simulink model "REALIZE_DISCRETE_LOOP_FILTER_L_z_WITHOUT_DELAY"  (R2025b)
settings: Solver=VariableStepAuto  StartTime=0.0  StopTime=100  RelTol=1e-3
libraries: dspsrcs4 x1
settings Model: Creator=Team_33  LastModifiedBy=k2vas

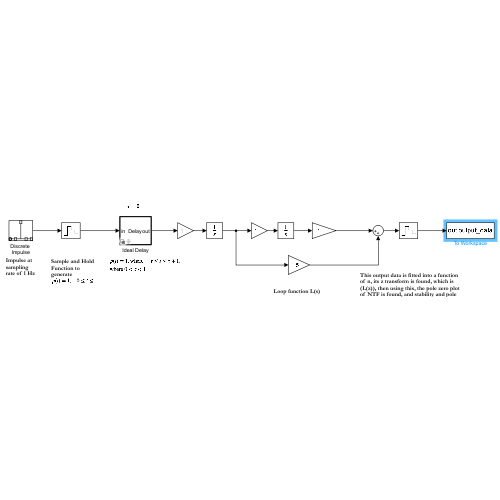
[thumbnail: Simulink's stored preview of the top-level diagram]
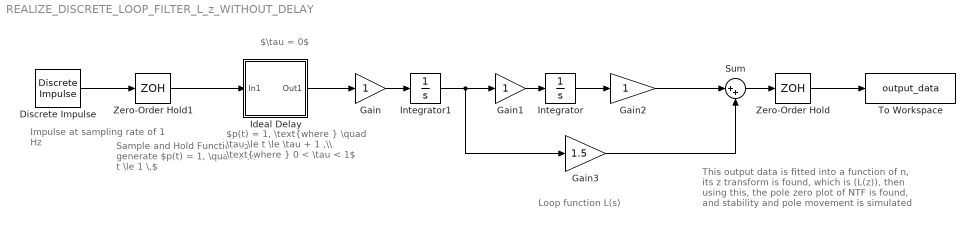
== system REALIZE_DISCRETE_LOOP_FILTER_L_z_WITHOUT_DELAY ==
  note: $\tau = 0$
  note: Sample and Hold Function to generate
      | $p(t) = 1, \quad 0 \le t \le 1 \,$
  note: $p(t) = 1, \text{where } \quad \tau \le t \le \tau + 1 ,\\ \text{where } 0 < \tau < 1$
  note: Impulse at sampling rate of 1 Hz
  note: Loop function L(s)
  note: This output data is fitted into a function of n, its z transform is found, which is (L(z)), then using this, the pole zero plot of NTF is found, and stability and pole movement is simulated
  Discrete Impulse : dspsrcs4/Discrete  Impulse  SFcnStateName=COUNT  Delay=0  SampleTime=1  FrameSample=1  OutputFrames=off  dataType=double  isSigned=on  wordLen=16  udDataType=sfix(16)  fracBitsMode=Best precision  numFracBits=15  OutDataTypeStr=double  LastOutDataTypeStr=double
      settings: SFcnIsStateOwnerBlock=on
  Gain : Gain
  Gain1 : Gain
  Gain2 : Gain
  Gain3 : Gain  Gain=1.5
  Ideal Delay : Subsystem  Variant=on  VariantControlMode=label  LabelModeActiveChoice=delayOFF  mask{eld=0, ts=1}
      mask prompts: eld "Excess delay"; ts "Sampling period"
      mask init:
      | eld = get_param(gcb, 'value@eld');
      |     if eld == 0
      |         set_param(gcb, 'LabelModeActiveChoice', 'delayOFF');
      |     else
      |         set_param(gcb, 'LabelModeActiveChoice', 'delayON');
      |     end
      mask Callback eld:
      | eld = get_param(gcb, 'value@eld');
      |     if eld == 0
      |         set_param(gcb, 'LabelModeActiveChoice', 'delayOFF');
      |     else
      |         set_param(gcb, 'LabelModeActiveChoice', 'delayON');
      |     end
      mask DialogControl DescTextVar Prompt: Ideal delay block (time delay = eld * Ts).
      mask Display:
      | plot([0 1 1 0 0], [0 0 1 1 0]);
      | text(0.5, 0.5, 'Delay', 'HorizontalAlignment','center', 'VerticalAlignment', 'middle');
      | port_label('input', 1, 'in');
      | port_label('output', 1, 'out');
  Integrator : Integrator
  Integrator1 : Integrator
  Sum : Sum  Inputs=|++
  To Workspace : ToWorkspace  VariableName=output_data  SampleTime=-1
      settings: Save2DSignal=2-D array (concatenate along first dimension)
  Zero-Order Hold : ZeroOrderHold
  Zero-Order Hold1 : ZeroOrderHold
  wires:
  Ideal Delay/1(Out1) -> Gain/1
  Gain2/1 -> Sum/1
  Gain3/1 -> Sum/2
  Gain/1 -> Integrator1/1
  Gain1/1 -> Integrator/1
  Integrator1/1 -> Gain3/1, Gain1/1
  Zero-Order Hold/1 -> To Workspace/1
  Integrator/1 -> Gain2/1
  Sum/1 -> Zero-Order Hold/1
  Discrete Impulse/1 -> Zero-Order Hold1/1
  Zero-Order Hold1/1 -> Ideal Delay/1(In1)

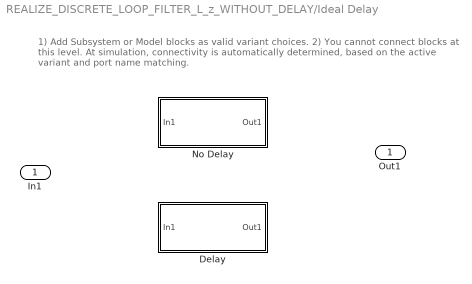
== system REALIZE_DISCRETE_LOOP_FILTER_L_z_WITHOUT_DELAY/Ideal Delay ==
  note: 1) Add Subsystem or Model blocks as valid variant choices.
      | 2) You cannot connect blocks at this level. At simulation, connectivity is automatically
      | determined, based on the active variant and port name matching.
  In1 : Inport
  Delay : Subsystem  VariantControl=delayON
  No Delay : Subsystem  VariantControl=delayOFF
  Out1 : Outport

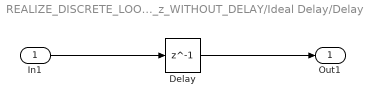
== system REALIZE_DISCRETE_LOOP_FILTER_L_z_WITHOUT_DELAY/Ideal Delay/Delay ==
  In1 : Inport
  Delay : Delay  DelayLength=1  SampleTime=eld*ts
  Out1 : Outport
  wires:
  Delay/1 -> Out1/1
  In1/1 -> Delay/1

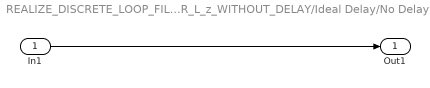
== system REALIZE_DISCRETE_LOOP_FILTER_L_z_WITHOUT_DELAY/Ideal Delay/No Delay ==
  In1 : Inport
  Out1 : Outport
  wires:
  In1/1 -> Out1/1
